simulink model "backups"  (R2024a)
settings: Solver=VariableStepAuto  StartTime=0.0  StopTime=10.0  RelTol=1e-3
values from neighbouring files (symbols this model uses):
  AttKd_x = inp(4,2).Var2    [SFF_Simulator_Entradas.m]
  AttKd_y = inp(5,2).Var2    [SFF_Simulator_Entradas.m]
  AttKd_z = inp(6,2).Var2    [SFF_Simulator_Entradas.m]
  AttKp_x = inp(1,2).Var2    [SFF_Simulator_Entradas.m]
  AttKp_y = inp(2,2).Var2    [SFF_Simulator_Entradas.m]
  AttKp_z = inp(3,2).Var2    [SFF_Simulator_Entradas.m]
  B = inp(8,2).Var2    [SFF_Simulator_Entradas.m]
  beta = inp(2,2).Var2    [SFF_Simulator_Entradas.m]
  Cd1 = inp(4,2).Var2    [SFF_Simulator_Entradas.m]
  cdgps = inp(1,2).Var2    [SFF_Simulator_Entradas.m]
  estrelas = inp(4,2).Var2    [SFF_Simulator_Entradas.m]
  estrelas_bias = inp(6,2).Var2    [SFF_Simulator_Entradas.m]
  estrelas_ruido = inp(5,2).Var2    [SFF_Simulator_Entradas.m]
  Fn = inp(2,2).Var2    [SFF_Simulator_Entradas.m]
  gps_bias = inp(3,2).Var2    [SFF_Simulator_Entradas.m]
  gps_ruido = inp(2,2).Var2    [SFF_Simulator_Entradas.m]
  Iw = inp(7,2).Var2    [SFF_Simulator_Entradas.m]
  Ixx = inp(7,2).Var2    [SFF_Simulator_Entradas.m]
  Iyy = inp(8,2).Var2    [SFF_Simulator_Entradas.m]
  Izz = inp(9,2).Var2    [SFF_Simulator_Entradas.m]
  Km = inp(3,2).Var2    [SFF_Simulator_Entradas.m]
  Kv = inp(9,2).Var2    [SFF_Simulator_Entradas.m]
  L1 = inp(5,2).Var2    [SFF_Simulator_Entradas.m]
  limCorrente = inp(4,2).Var2    [SFF_Simulator_Entradas.m]
  limVolt = inp(5,2).Var2    [SFF_Simulator_Entradas.m]
  m1 = inp(6,2).Var2    [SFF_Simulator_Entradas.m]
  magne = inp(10,2).Var2    [SFF_Simulator_Entradas.m]
  magne_bias = inp(12,2).Var2    [SFF_Simulator_Entradas.m]
  magne_ruido = inp(11,2).Var2    [SFF_Simulator_Entradas.m]
  man = inp(1,2).Var2    [SFF_Simulator_Entradas.m]
  OrbKd_x = inp(3,2).Var2    [SFF_Simulator_Entradas.m]
  OrbKd_y = inp(6,2).Var2    [SFF_Simulator_Entradas.m]
  OrbKd_z = inp(9,2).Var2    [SFF_Simulator_Entradas.m]
  OrbKi_x = inp(2,2).Var2    [SFF_Simulator_Entradas.m]
  OrbKi_y = inp(5,2).Var2    [SFF_Simulator_Entradas.m]
  OrbKi_z = inp(8,2).Var2    [SFF_Simulator_Entradas.m]
  OrbKp_x = inp(1,2).Var2    [SFF_Simulator_Entradas.m]
  OrbKp_y = inp(4,2).Var2    [SFF_Simulator_Entradas.m]
  OrbKp_z = inp(7,2).Var2    [SFF_Simulator_Entradas.m]
  propForcaAtivo = inp(1,2).Var2    [SFF_Simulator_Entradas.m]
  Rm = inp(6,2).Var2    [SFF_Simulator_Entradas.m]
  rodaAtivo = inp(1,2).Var2    [SFF_Simulator_Entradas.m]
  RodKi = inp(1,2).Var2    [SFF_Simulator_Entradas.m]
  sat_torquerod = inp(14,2).Var2    [SFF_Simulator_Entradas.m]
  torqrodAtivo = inp(1,2).Var2    [SFF_Simulator_Entradas.m]
undefined symbols (not defined in the file or in its folder): IAU, J2, mi, omega_E, propMomentoAtivo, Re, sat_rodareacao, WMM2020
libraries: dspsrcs4 x19, aerolibtransform2 x2, aerolibgravity2 x2, simulink x1
(part 4 of 4)

== system backups/Atuadores de Atitude/Atuador atitude ativado/Magnetorquer ativado/Magnetômetro/If Action Subsystem/magneSensor ==
  In1 : Inport
  Add1 : Sum
  Add2 : Sum
  Constant : Constant  Value=magne_bias
  Random Source1 : dspsrcs4/Random Source  SrcType=Uniform  MinVal=-magne_ruido  MaxVal=magne_ruido  MeanVal=0  VarVal=1  RepMode=Not repeatable  rawSeed=1  IsInherit=off  SampTime=step_modelo  SampFrame=1  OutComplex=Real  DataType=double  SimulateUsing=Code generation
  Out1 : Outport
  wires:
  Random Source1/1 -> Add2/1
  In1/1 -> Add1/2
  Constant/1 -> Add1/1
  Add1/1 -> Add2/2
  Add2/1 -> Out1/1

== system backups/Atuadores de Atitude/Atuador atitude ativado/Magnetorquer ativado/Magnetômetro/If Action Subsystem/magneSensor1 ==
  In1 : Inport
  Add1 : Sum
  Add2 : Sum
  Constant : Constant  Value=magne_bias
  Random Source1 : dspsrcs4/Random Source  SrcType=Uniform  MinVal=-magne_ruido  MaxVal=magne_ruido  MeanVal=0  VarVal=1  RepMode=Not repeatable  rawSeed=1  IsInherit=off  SampTime=step_modelo  SampFrame=1  OutComplex=Real  DataType=double  SimulateUsing=Code generation
  Out1 : Outport
  wires:
  Add2/1 -> Out1/1
  Add1/1 -> Add2/2
  Random Source1/1 -> Add2/1
  In1/1 -> Add1/2
  Constant/1 -> Add1/1

== system backups/Atuadores de Atitude/Atuador atitude ativado/Magnetorquer ativado/Magnetômetro/If Action Subsystem/magneSensor2 ==
  In1 : Inport
  Add1 : Sum
  Add2 : Sum
  Constant : Constant  Value=magne_bias
  Random Source1 : dspsrcs4/Random Source  SrcType=Uniform  MinVal=-magne_ruido  MaxVal=magne_ruido  MeanVal=0  VarVal=1  RepMode=Not repeatable  rawSeed=1  IsInherit=off  SampTime=step_modelo  SampFrame=1  OutComplex=Real  DataType=double  SimulateUsing=Code generation
  Out1 : Outport
  wires:
  Add2/1 -> Out1/1
  Add1/1 -> Add2/2
  Random Source1/1 -> Add2/1
  In1/1 -> Add1/2
  Constant/1 -> Add1/1

== system backups/Atuadores de Atitude1/Atuador atitude ativado/Magnetorquer ativado/Magnetômetro/If Action Subsystem/magneSensor ==
  In1 : Inport
  Add1 : Sum
  Add2 : Sum
  Constant : Constant  Value=magne_bias
  Random Source1 : dspsrcs4/Random Source  SrcType=Uniform  MinVal=-magne_ruido  MaxVal=magne_ruido  MeanVal=0  VarVal=1  RepMode=Not repeatable  rawSeed=1  IsInherit=off  SampTime=step_modelo  SampFrame=1  OutComplex=Real  DataType=double  SimulateUsing=Code generation
  Out1 : Outport
  wires:
  Random Source1/1 -> Add2/1
  In1/1 -> Add1/2
  Constant/1 -> Add1/1
  Add1/1 -> Add2/2
  Add2/1 -> Out1/1

== system backups/Atuadores de Atitude1/Atuador atitude ativado/Magnetorquer ativado/Magnetômetro/If Action Subsystem/magneSensor1 ==
  In1 : Inport
  Add1 : Sum
  Add2 : Sum
  Constant : Constant  Value=magne_bias
  Random Source1 : dspsrcs4/Random Source  SrcType=Uniform  MinVal=-magne_ruido  MaxVal=magne_ruido  MeanVal=0  VarVal=1  RepMode=Not repeatable  rawSeed=1  IsInherit=off  SampTime=step_modelo  SampFrame=1  OutComplex=Real  DataType=double  SimulateUsing=Code generation
  Out1 : Outport
  wires:
  Add2/1 -> Out1/1
  Add1/1 -> Add2/2
  Random Source1/1 -> Add2/1
  In1/1 -> Add1/2
  Constant/1 -> Add1/1

== system backups/Atuadores de Atitude1/Atuador atitude ativado/Magnetorquer ativado/Magnetômetro/If Action Subsystem/magneSensor2 ==
  In1 : Inport
  Add1 : Sum
  Add2 : Sum
  Constant : Constant  Value=magne_bias
  Random Source1 : dspsrcs4/Random Source  SrcType=Uniform  MinVal=-magne_ruido  MaxVal=magne_ruido  MeanVal=0  VarVal=1  RepMode=Not repeatable  rawSeed=1  IsInherit=off  SampTime=step_modelo  SampFrame=1  OutComplex=Real  DataType=double  SimulateUsing=Code generation
  Out1 : Outport
  wires:
  Add2/1 -> Out1/1
  Add1/1 -> Add2/2
  Random Source1/1 -> Add2/1
  In1/1 -> Add1/2
  Constant/1 -> Add1/1

== system backups/atuadoresAtitude/conjunto2TorqRods1RodaReacao/HardwareDeControle (Rodas de Reação + 2 Torqrods)/rodaReacaoCaracteristicas/Subsystem/Controlador Integral ==
  Erro na corrente : Inport
  Gain : Gain  Gain=RodKi
  Integrator : Integrator
  Voltagem : Outport  VectorParamsAs1DForOutWhenUnconnected=off
  wires:
  Gain/1 -> Integrator/1
  Erro na corrente/1 -> Gain/1
  Integrator/1 -> Voltagem/1

== matlab function backups/dinamicaCinematicaAtitude1/MATLAB Function ==
  data: u input; phi output; theta output; psi output
function [phi,theta,psi] = fcn(u)

y = quat2eul([u(4) u(1) u(2) u(3)]);

phi = y(1);
theta = y(2);
psi = y(3);

== matlab function backups/errosAngAtitude1/MATLAB Function4 ==
  data: q_d input; q_error output; q input
function q_error = fcn(q_d,q)

qt1 = q_d(1);
qt2 = q_d(2);
qt3 = q_d(3);
qt4 = q_d(4);

qs1 = q(1);
qs2 = q(2);
qs3 = q(3);
qs4 = q(4);

% q_error = [qt4 qt3 -qt2 -qt1
%     -qt3 qt4 qt1 -qt2
%     qt2 -qt1 qt4 -qt3
%     qt1 qt2 qt3 qt4]*[qs1;qs2;qs3;qs4];

q_error = [qt4 qt3 -qt2 qt1
    -qt3 qt4 qt1 qt2
    qt2 -qt1 qt4 qt3
    -qt1 -qt2 -qt3 qt4]*[-qs1;-qs2;-qs3;qs4];

== matlab function backups/Atuadores Orbital/forçasSistCorpoSeg ==
  data: A_q input; Fx_b output; m1 input; controleOrbital input; Fy_b output; Fz_b output
function [Fx_b,Fy_b,Fz_b] = fcn(A_q,m1,controleOrbital)

ux = controleOrbital(1);
uy = controleOrbital(2);
uz = controleOrbital(3);

Fx = m1*ux;
Fy = m1*uy;
Fz = m1*uz;

F_b = A_q*[Fx; Fy; Fz];

Fx_b = F_b(1);
Fy_b = F_b(2);
Fz_b = F_b(3);

== matlab function backups/Atuadores de Atitude/Atuador atitude ativado/Magnetorquer ativado/Conjunto Rodas de Reação + Magnetotorques/B_matriz ==
  data: B_seg input; y output
function y = fcn(B_seg)

Bx = B_seg(1);
By = B_seg(2);
Bz = B_seg(3);

y = [0 0 -By
    -Bz 1 Bx
    By 0 0];

== matlab function backups/Atuadores de Atitude/Atuador atitude ativado/Magnetorquer ativado/Conjunto Rodas de Reação + Magnetotorques/Inv_B_matriz ==
  data: B_seg input; y output
function y = fcn(B_seg)

Bx = B_seg(1);
By = B_seg(2);
Bz = B_seg(3);

if By == 0
    y = [0 0 0; 0 0 0; 0 0 0];
else
    y = (1/(By^2))*[0 0 By
    Bx*By By^2 By*Bz
    -By 0 0];
end

== matlab function backups/Dinâmica Cinemática Atitude/MATLAB Function ==
  data: u input; phi output; theta output; psi output
function [phi,theta,psi] = fcn(u)

y = quat2eul([u(4) u(1) u(2) u(3)]);

phi = wrapToPi(y(1));
theta = wrapToPi(y(2));
psi = wrapToPi(y(3));

== matlab function backups/Erros Quatérnions/MATLAB Function4 ==
  data: q_d input; q_error output; q input
function q_error = fcn(q_d,q)

qt1 = q_d(1);
qt2 = q_d(2);
qt3 = q_d(3);
qt4 = q_d(4);

qs1 = q(1);
qs2 = q(2);
qs3 = q(3);
qs4 = q(4);

q_error = [qt4 qt3 -qt2 qt1
    -qt3 qt4 qt1 qt2
    qt2 -qt1 qt4 qt3
    -qt1 -qt2 -qt3 qt4]*[-qs1;-qs2;-qs3;qs4];

== matlab function backups/Guiamento Atitude/Euler -> Quatérnions ==
  data: phi_ref input; q_ref output; theta_ref input; psi_ref input
function q_ref = fcn(phi_ref,theta_ref,psi_ref)

q_ref = eul2quat([phi_ref theta_ref psi_ref]);

q_ref = [q_ref(2),q_ref(3),q_ref(4),q_ref(1)];

== matlab function backups/GuiamentoAtitude/Euler -> Quatérnions ==
  data: phi_ref input; q_ref output; theta_ref input; psi_ref input
function q_ref = fcn(phi_ref,theta_ref,psi_ref)

q_ref = eul2quat([phi_ref theta_ref psi_ref]);

q_ref = [q_ref(2),q_ref(3),q_ref(4),q_ref(1)];

== matlab function backups/Sensores Atitude/Euler -> Quat ==
  data: phi_ref input; q_ref output; theta_ref input; psi_ref input; q_in input
function q_ref = fcn(phi_ref,theta_ref,psi_ref,q_in)

q_ref = eul2quat([phi_ref theta_ref psi_ref]);

q_ref = [sign(q_in(1))*abs(q_ref(2)),sign(q_in(2))*abs(q_ref(3)),sign(q_in(3))*abs(q_ref(4)),sign(q_in(4))*abs(q_ref(1))];

== matlab function backups/Sensores Atitude/Quat -> Euler ==
  data: u input; phi output; theta output; psi output
function [phi,theta,psi] = fcn(u)

y = quat2eul([u(4) u(1) u(2) u(3)]);

phi = (y(1)); 
theta = (y(2));
psi = (y(3));

== matlab function backups/Atuadores Orbital1/acelSistLVLHSeg1 ==
  data: A_q input; acelx output; m1 input; F_b input; acely output; acelz output
function [acelx,acely,acelz] = fcn(A_q,m1,F_b)

F_real = A_q'*F_b;

Fx_real = F_real(1);
Fy_real = F_real(2);
Fz_real = F_real(3);


acelx = Fx_real/m1;
acely = Fy_real/m1;
acelz = Fz_real/m1;

== matlab function backups/Atuadores Orbital1/forçasSistCorpoSeg ==
  data: A_q input; Fx_b output; m1 input; controleOrbital input; Fy_b output; Fz_b output
function [Fx_b,Fy_b,Fz_b] = fcn(A_q,m1,controleOrbital)

ux = controleOrbital(1);
uy = controleOrbital(2);
uz = controleOrbital(3);

Fx = m1*ux;
Fy = m1*uy;
Fz = m1*uz;

F_b = A_q*[Fx; Fy; Fz];

Fx_b = F_b(1);
Fy_b = F_b(2);
Fz_b = F_b(3);

== matlab function backups/Atuadores de Atitude1/Atuador atitude ativado/Magnetorquer ativado/HardwareDeControle (Rodas de Reação + 2 Torqrods)/B_matriz ==
  data: B_seg input; y output
function y = fcn(B_seg)

Bx = B_seg(1);
By = B_seg(2);
Bz = B_seg(3);

y = [0 0 -By
    -Bz 1 Bx
    By 0 0];

== matlab function backups/Atuadores de Atitude1/Atuador atitude ativado/Magnetorquer ativado/HardwareDeControle (Rodas de Reação + 2 Torqrods)/Inv_B_matriz ==
  data: B_seg input; y output
function y = fcn(B_seg)

Bx = B_seg(1);
By = B_seg(2);
Bz = B_seg(3);

if By == 0
    y = [0 0 0; 0 0 0; 0 0 0];
else
    y = (1/(By^2))*[0 0 By
    Bx*By By^2 By*Bz
    -By 0 0];
end

== matlab function backups/Dinâmica Cinemática Atitude1/MATLAB Function ==
  data: u input; phi output; theta output; psi output
function [phi,theta,psi] = fcn(u)

y = quat2eul([u(4) u(1) u(2) u(3)]);

phi = wrapToPi(y(1));
theta = wrapToPi(y(2));
psi = wrapToPi(y(3));

== matlab function backups/Erros Quatérnions1/MATLAB Function4 ==
  data: q_d input; q_error output; q input
function q_error = fcn(q_d,q)

qt1 = q_d(1);
qt2 = q_d(2);
qt3 = q_d(3);
qt4 = q_d(4);

qs1 = q(1);
qs2 = q(2);
qs3 = q(3);
qs4 = q(4);

q_error = [qt4 qt3 -qt2 qt1
    -qt3 qt4 qt1 qt2
    qt2 -qt1 qt4 qt3
    -qt1 -qt2 -qt3 qt4]*[-qs1;-qs2;-qs3;qs4];

== matlab function backups/Guiamento Atitude1/Euler -> Quatérnions ==
  data: phi_ref input; q_ref output; theta_ref input; psi_ref input
function q_ref = fcn(phi_ref,theta_ref,psi_ref)

q_ref = eul2quat([phi_ref theta_ref psi_ref]);

q_ref = [q_ref(2),q_ref(3),q_ref(4),q_ref(1)];

== matlab function backups/Sensores Atitude1/Euler -> Quatérnions ==
  data: phi_ref input; q_ref output; theta_ref input; psi_ref input; q_in input
function q_ref = fcn(phi_ref,theta_ref,psi_ref,q_in)

q_ref = eul2quat([phi_ref theta_ref psi_ref]);

q_ref = [sign(q_in(1))*abs(q_ref(2)),sign(q_in(2))*abs(q_ref(3)),sign(q_in(3))*abs(q_ref(4)),sign(q_in(4))*abs(q_ref(1))];

== matlab function backups/atuadoresAtitude/MATLAB Function ==
  data: propMomentoAtivo input; y output; rodaAtivo input; torqrodAtivo input; Mts input; u1 input; u2 input; u3 input
function y = fcn(propMomentoAtivo,rodaAtivo,torqrodAtivo,Mts,u1,u2,u3)


if propMomentoAtivo
    y = u1;
elseif rodaAtivo
    y = u2;
elseif torqrodAtivo
    y = u3;
else    
    y = Mts;
end

== matlab function backups/Sensores Atitude1/quat>euler ==
  data: u input; phi output; theta output; psi output
function [phi,theta,psi] = fcn(u)

y = quat2eul([u(4) u(1) u(2) u(3)]);

phi = (y(1)); 
theta = (y(2));
psi = (y(3));

== matlab function backups/wrapTo2Pi1 ==
  data: u input; y output
function y = fcn(u)



y = wrapTo2Pi(u);

== matlab function backups/atuadoresAtitude/conjunto2TorqRods1RodaReacao/HardwareDeControle (Rodas de Reação + 2 Torqrods)/B_matriz ==
  data: B_seg input; y output
function y = fcn(B_seg)

Bx = B_seg(1);
By = B_seg(2);
Bz = B_seg(3);

y = [0 0 -By
    -Bz 1 Bx
    By 0 0];

== matlab function backups/forçasSistCorpoSeg1 ==
  data: A_q input; Fx_b output; m1 input; controleOrbital input; Fy_b output; Fz_b output
function [Fx_b,Fy_b,Fz_b] = fcn(A_q,m1,controleOrbital)

ux = controleOrbital(1);
uy = controleOrbital(2);
uz = controleOrbital(3);

Fx = m1*ux;
Fy = m1*uy;
Fz = m1*uz;

F_b = A_q*[Fx; Fy; Fz];

Fx_b = F_b(1);
Fy_b = F_b(2);
Fz_b = F_b(3);

== matlab function backups/atuadoresAtitude/conjunto2TorqRods1RodaReacao/HardwareDeControle (Rodas de Reação + 2 Torqrods)/Inv_B_matriz ==
  data: B_seg input; y output
function y = fcn(B_seg)

Bx = B_seg(1);
By = B_seg(2);
Bz = B_seg(3);

if By == 0
    y = [0 0 0; 0 0 0; 0 0 0];
else
    y = (1/(By^2))*[0 0 By
    Bx*By By^2 By*Bz
    -By 0 0];
end

== matlab function backups/atuadoresOrbital1/acelSistLVLHSeg1 ==
  data: A_q input; acelx output; m1 input; F_b input; acely output; acelz output
function [acelx,acely,acelz] = fcn(A_q,m1,F_b)

F_real = A_q'*F_b;

Fx_real = F_real(1);
Fy_real = F_real(2);
Fz_real = F_real(3);


acelx = Fx_real/m1;
acely = Fy_real/m1;
acelz = Fz_real/m1;

== matlab function backups/Atuadores Orbital/acelSistLVLHSeg1 ==
  data: A_q input; acelx output; m1 input; F_b input; acely output; acelz output
function [acelx,acely,acelz] = fcn(A_q,m1,F_b)

F_real = A_q'*F_b;

Fx_real = F_real(1);
Fy_real = F_real(2);
Fz_real = F_real(3);


acelx = Fx_real/m1;
acely = Fy_real/m1;
acelz = Fz_real/m1;

== matlab function backups/atuadoresOrbital1/forçasSistCorpoSeg ==
  data: A_q input; Fx_b output; m1 input; controleOrbital input; Fy_b output; Fz_b output
function [Fx_b,Fy_b,Fz_b] = fcn(A_q,m1,controleOrbital)

ux = controleOrbital(1);
uy = controleOrbital(2);
uz = controleOrbital(3);

Fx = m1*ux;
Fy = m1*uy;
Fz = m1*uz;

F_b = A_q*[Fx; Fy; Fz];

Fx_b = F_b(1);
Fy_b = F_b(2);
Fz_b = F_b(3);
